simulink model "Filtro1"  (R2021b)
settings: Solver=VariableStepAuto  StartTime=0.0  StopTime=10.0  RelTol=1e-3
settings Model: Creator=cesar  LastModifiedBy=cesar

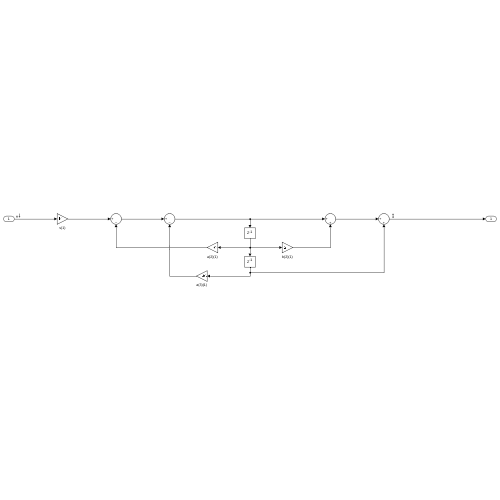
[thumbnail: Simulink's stored preview of the top-level diagram]
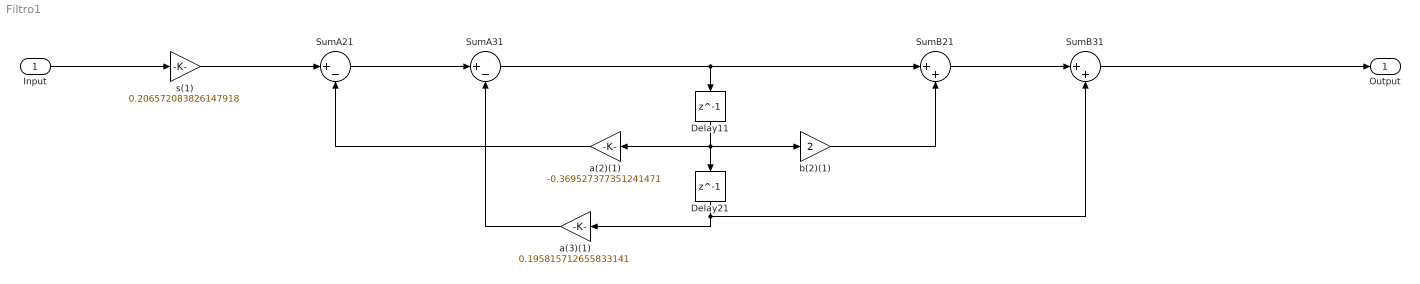
== system Filtro1 ==
  Input : Inport
  Delay11 : Delay  DelayLength=1  InitialCondition=0
  Delay21 : Delay  DelayLength=1  InitialCondition=0
  SumA21 : Sum  Inputs=|+-  RndMeth=Nearest  SaturateOnIntegerOverflow=on  OutDataTypeStr=Inherit: Same as first input
  SumA31 : Sum  Inputs=|+-  RndMeth=Nearest  SaturateOnIntegerOverflow=on  OutDataTypeStr=Inherit: Same as first input
  SumB21 : Sum  Inputs=|++  RndMeth=Nearest  SaturateOnIntegerOverflow=on  OutDataTypeStr=Inherit: Same as first input
  SumB31 : Sum  Inputs=|++  RndMeth=Nearest  SaturateOnIntegerOverflow=on  OutDataTypeStr=Inherit: Same as first input
  a(2)(1) : Gain  Gain=-0.369527377351241471  ParamDataTypeStr=double  RndMeth=Nearest  SaturateOnIntegerOverflow=on  OutDataTypeStr=Inherit: Same as input
  a(3)(1) : Gain  Gain=0.195815712655833141  ParamDataTypeStr=double  RndMeth=Nearest  SaturateOnIntegerOverflow=on  OutDataTypeStr=Inherit: Same as input
  b(2)(1) : Gain  Gain=2  ParamDataTypeStr=double  RndMeth=Nearest  SaturateOnIntegerOverflow=on  OutDataTypeStr=Inherit: Same as input
  s(1) : Gain  Gain=0.206572083826147918  ParamDataTypeStr=double  RndMeth=Nearest  SaturateOnIntegerOverflow=on  OutDataTypeStr=Inherit: Same as input
  Output : Outport
  wires:
  SumB31/1 -> Output/1
  s(1)/1 -> SumA21/1
  SumA31/1 -> SumB21/1, Delay11/1
  Delay11/1 -> a(2)(1)/1, b(2)(1)/1, Delay21/1
  a(3)(1)/1 -> SumA31/2
  Input/1 -> s(1)/1
  Delay21/1 -> a(3)(1)/1, SumB31/2
  b(2)(1)/1 -> SumB21/2
  a(2)(1)/1 -> SumA21/2
  SumA21/1 -> SumA31/1
  SumB21/1 -> SumB31/1
